simulink model "meart_host_60"  (Simulink 6.5)
settings: Solver=FixedStepDiscrete  StartTime=0.0  StopTime=Inf  RelTol=1e-3
values from neighbouring files (symbols this model uses):
  threshold = -10*std(data)    [setthresh.m]
libraries: simulink x9, xpclib x5, dspindex x4, dspsigops x2, dspstat3 x1
settings Model: Creator=adowd  LastModifiedBy=avnerw
settings OptimizationCC: InlineInvariantSignals=on
settings DebuggingCC: MultiTaskDSMMsg=warning  MultiTaskCondExecSysMsg=none  StrictBusMsg=None
settings RTWCC: IncludeERTFirstTime=on

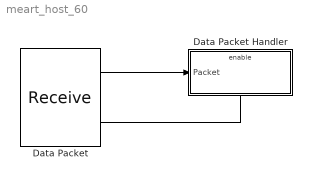
== system meart_host_60 ==
  Data Packet : xpclib/UDP/Receive  ipAddress=192.168.0.10  ipPort=25000  width=5524  sampletime=0.0008
  Data Packet Handler : Subsystem  TreatAsAtomicUnit=on
  wires:
  Data Packet/1 -> Data Packet Handler/1(Packet)
  Data Packet/2 -> Data Packet Handler/Enable

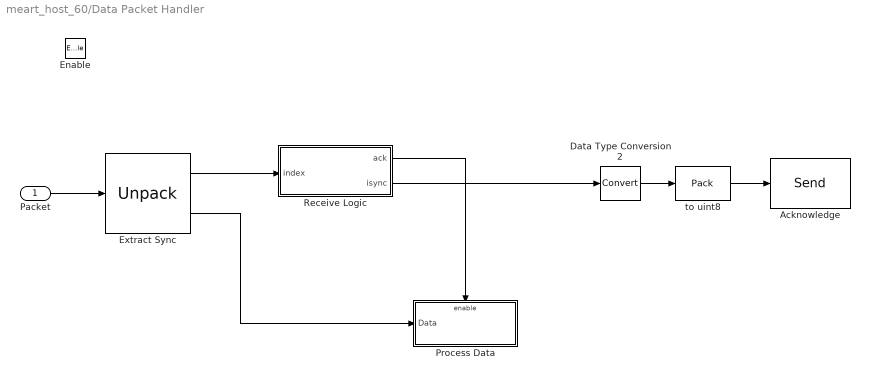
== system meart_host_60/Data Packet Handler ==
  Packet : Inport
  Enable : EnablePort
  Acknowledge : xpclib/UDP/Send  ipAddress=192.168.0.10  ipPort=25001  localPort=-1  sampletime=-1
  Data Type Conversion2 : DataTypeConversion  OutDataTypeMode=uint32
  Extract Sync : xpclib/UDP/Unpack  dimensions={1,5520}  datatypes={'uint32','uint8'}  byteAlign=1
  Process Data : Subsystem  TreatAsAtomicUnit=on
  Receive Logic : Stateflow chart
  to uint8 : xpclib/UDP/Pack  datatypes={'uint32'}  byteAlign=1
  wires:
  to uint8/1 -> Acknowledge/1
  Data Type Conversion2/1 -> to uint8/1
  Receive Logic/1(ack) -> Process Data/Enable
  Receive Logic/2(isync) -> Data Type Conversion2/1
  Extract Sync/1 -> Receive Logic/1(index)
  Extract Sync/2 -> Process Data/1(Data)
  Packet/1 -> Extract Sync/1

== system meart_host_60/Data Packet Handler/Process Data ==
  Data : Inport
  Enable : EnablePort
  Iterate Frames : Subsystem  TreatAsAtomicUnit=on
  Reshape : Reshape  OutputDimensionality=Customize (N-D)  OutputDimensions=[552,10]
  wires:
  Data/1 -> Reshape/1
  Reshape/1 -> Iterate Frames/1(Data Packet)

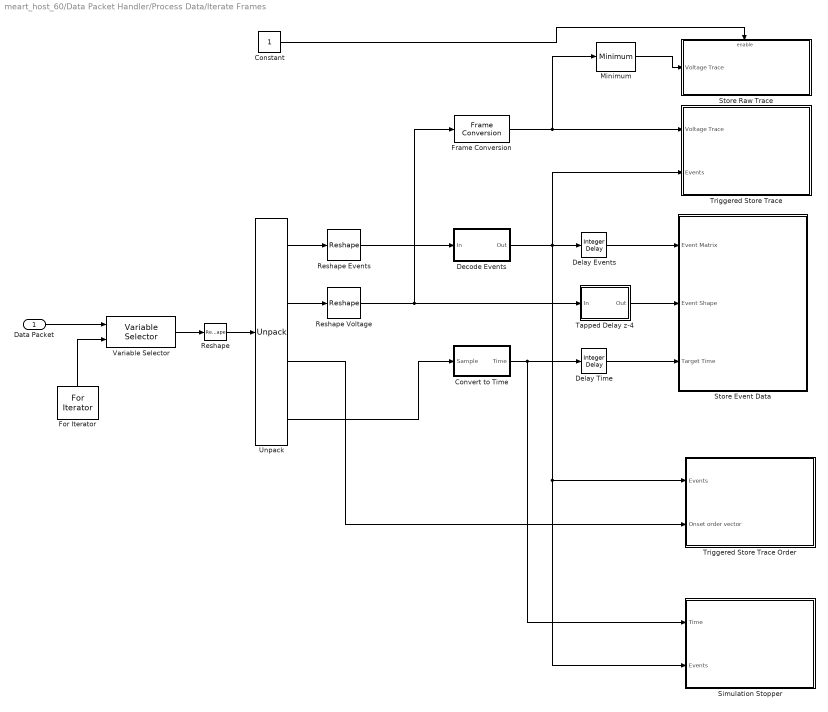
== system meart_host_60/Data Packet Handler/Process Data/Iterate Frames ==
  Data Packet : Inport
  Constant : Constant  Value=1  OutDataType=sfix(16)  ConRadixGroup=Use specified scaling  OutScaling=2^0  SampleTime=inf  FramePeriod=inf
  Convert to Time : Subsystem  mask{frametime=0.0005}
      mask prompts: frametime "Frametime (s):"
  Decode Events : Subsystem
  Delay Events : simulink/Discrete/Integer Delay  vinit=0  samptime=-1  NumDelays=3
  Delay Time : simulink/Discrete/Integer Delay  vinit=0  samptime=-1  NumDelays=3
  For Iterator : ForIterator  Orientation=up  IterationLimit=10  IterationVariableDataType=int16
  Frame Conversion : FrameConversion
  Minimum : dspstat3/Minimum  DialogController=dspfixptddg.MinMax  DialogControllerArgs=DataTag0  fcn=Value  reset=None  indexBase=One  operateOver=Each column  colComp=on  operation=minimum  roundingMode=Floor  overflowMode=off
  Reshape : Reshape
  Reshape Events : Reshape  OutputDimensionality=Customize (N-D)  OutputDimensions=[1,2]
  Reshape Voltage : Reshape  OutputDimensionality=Customize (N-D)  OutputDimensions=[8,60]
  Simulation Stopper : Subsystem  TreatAsAtomicUnit=on  mask{maxtrigs=10000, triggerchannel=61, delayframes=15*2}
      mask prompts: maxtrigs "Maximum number of triggers to concatenate:"; triggerchannel "Trigger to Channel:"; delayframes "Number of frames to delay before stopping the hosr after last trig"
  Store Event Data : Subsystem  TreatAsAtomicUnit=on
  Store Raw Trace : Subsystem  TreatAsAtomicUnit=on  mask{maxsamples=2000*3}
      mask prompts: maxsamples "Maximum number of samples  to concatenate:"
  Tapped Delay z-4 : Subsystem
  Triggered Store Trace : Subsystem  TreatAsAtomicUnit=on  mask{presamples=0, postsamples=15*2, maxrecords=3600, triggerchannel=61}
      mask prompts: presamples "Presamples (frames):"; postsamples "Postsamples (frames):"; maxrecords "Maximum number of records to concatenate:"; triggerchannel "Trigger to Channel:"
  Triggered Store Trace Order : Subsystem  TreatAsAtomicUnit=on  mask{offsettimeframes=15*2, maxrecords=10000, triggerchannel=61}
      mask prompts: offsettimeframes "offset time (frames):"; maxrecords "Maximum number of records to concatenate:"; triggerchannel "Trigger to Channel:"
  Unpack : xpclib/UDP/Unpack  dimensions={2, 480,60, 1}  datatypes={'uint32', 'int8', 'uint8','uint32'}  byteAlign=1
  Variable Selector : dspindex/Variable Selector  NumInputs=1  rowsOrCols=Columns  IdxMode=Variable  Elements=[1 3]  ZerOneIdxMode=One-based  errmode=Generate Error  FillMode=off  FillValues=0
  wires:
  Unpack/2 -> Reshape Voltage/1
  Unpack/1 -> Reshape Events/1
  Reshape Events/1 -> Decode Events/1(In)
  Decode Events/1(Out) -> Triggered Store Trace/2(Events), Delay Events/1, Triggered Store Trace Order/1(Events), Simulation Stopper/2(Events)
  Reshape Voltage/1 -> Frame Conversion/1, Tapped Delay z-4/1(In)
  Data Packet/1 -> Variable Selector/1
  For Iterator/1 -> Variable Selector/2
  Variable Selector/1 -> Reshape/1
  Reshape/1 -> Unpack/1
  Frame Conversion/1 -> Triggered Store Trace/1(Voltage Trace), Minimum/1
  Minimum/1 -> Store Raw Trace/1(Voltage Trace)
  Convert to Time/1(Time) -> Delay Time/1, Simulation Stopper/1(Time)
  Delay Time/1 -> Store Event Data/3(Target Time)
  Delay Events/1 -> Store Event Data/1(Event Matrix)
  Tapped Delay z-4/1(Out) -> Store Event Data/2(Event Shape)
  Constant/1 -> Store Raw Trace/Enable
  Unpack/4 -> Convert to Time/1(Sample)
  Unpack/3 -> Triggered Store Trace Order/2(Onset order vector)

== system meart_host_60/Data Packet Handler/Process Data/Iterate Frames/Convert to Time ==
  Sample : Inport
  Convert Seconds : Product  Inputs=**  OutDataTypeMode=double  OutScaling=2^-10
  Frametime : Constant  Orientation=up  Value=frametime  OutDataTypeMode=double  OutDataType=sfix(16)  ConRadixGroup=Use specified scaling  OutScaling=2^0  SampleTime=inf  FramePeriod=inf
  Time : Outport
  wires:
  Convert Seconds/1 -> Time/1
  Frametime/1 -> Convert Seconds/2
  Sample/1 -> Convert Seconds/1

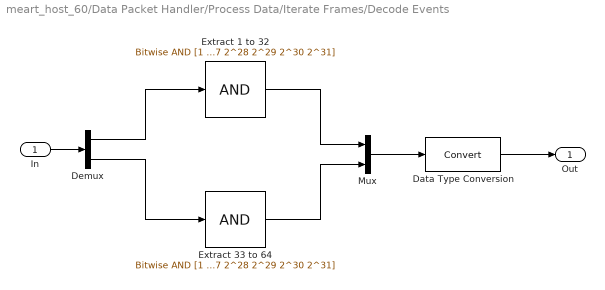
== system meart_host_60/Data Packet Handler/Process Data/Iterate Frames/Decode Events ==
  In : Inport  PortDimensions=2  DataType=uint32
  Data Type Conversion : DataTypeConversion  OutDataTypeMode=boolean
  Demux : Demux  Outputs=2
  Extract 1 to 32 : simulink/Logic and Bit Operations/Bitwise Operator  logicop=AND  UseBitMask=on  BitMask=[1 2 2^2 2^3 2^4 2^5 2^6 2^7 2^8 2^9 2^10 2^11 2^12 2^13 2^14 2^15 2^16 2^17 2^18 2^19 2^20 2^21 2^22 2^23 2^24 2^25 2^26 2^27 2^28 2^29 2^30 2^31]  BitMaskRealWorld=Stored Integer
  Extract 33 to 64 : simulink/Logic and Bit Operations/Bitwise Operator  logicop=AND  UseBitMask=on  BitMask=[1 2 2^2 2^3 2^4 2^5 2^6 2^7 2^8 2^9 2^10 2^11 2^12 2^13 2^14 2^15 2^16 2^17 2^18 2^19 2^20 2^21 2^22 2^23 2^24 2^25 2^26 2^27 2^28 2^29 2^30 2^31]  BitMaskRealWorld=Stored Integer
  Mux : Mux  Inputs=2
  Out : Outport  DataType=boolean
  wires:
  In/1 -> Demux/1
  Demux/1 -> Extract 1 to 32/1
  Demux/2 -> Extract 33 to 64/1
  Extract 33 to 64/1 -> Mux/2
  Mux/1 -> Data Type Conversion/1
  Data Type Conversion/1 -> Out/1
  Extract 1 to 32/1 -> Mux/1

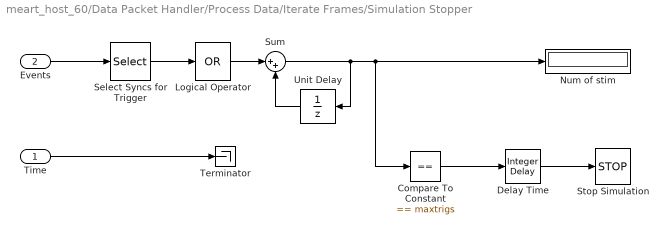
== system meart_host_60/Data Packet Handler/Process Data/Iterate Frames/Simulation Stopper ==
  Time : Inport
  Events : Inport  Port=2
  Compare To Constant : simulink/Logic and Bit Operations/Compare To Constant  SystemSampleTime=-1  relop===  const=maxtrigs  LogicOutDataTypeMode=boolean  ZeroCross=off
  Delay Time : simulink/Discrete/Integer Delay  vinit=0  samptime=-1  NumDelays=delayframes
  Logical Operator : Logic  Operator=OR  Inputs=1  AllPortsSameDT=off  OutDataTypeMode=Boolean
  Num of stim : Display
  Select Syncs for Trigger : Selector  InputType=Vector  ElementSrc=Internal  Elements=triggerchannel  RowSrc=Internal  Rows=1  ColumnSrc=Internal  Columns=1  InputPortWidth=64  IndexIsStartValue=off
  Stop Simulation : Stop
  Sum : Sum  Inputs=|++  OutDataTypeMode=double
  Terminator : Terminator
  Unit Delay : UnitDelay  Orientation=left  SampleTime=-1
  wires:
  Time/1 -> Terminator/1
  Select Syncs for Trigger/1 -> Logical Operator/1
  Events/1 -> Select Syncs for Trigger/1
  Sum/1 -> Compare To Constant/1, Num of stim/1, Unit Delay/1
  Compare To Constant/1 -> Delay Time/1
  Unit Delay/1 -> Sum/2
  Logical Operator/1 -> Sum/1
  Delay Time/1 -> Stop Simulation/1

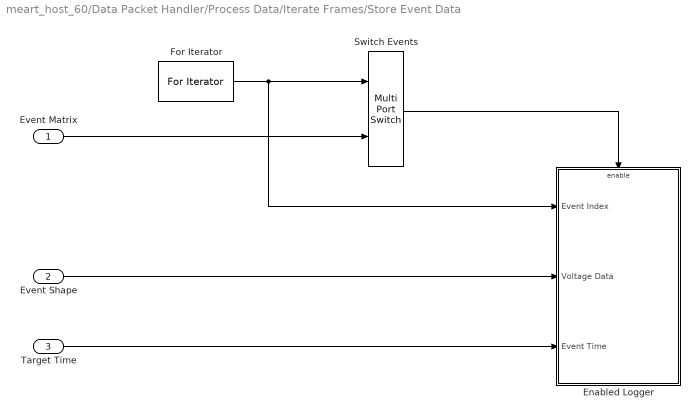
== system meart_host_60/Data Packet Handler/Process Data/Iterate Frames/Store Event Data ==
  Event Matrix : Inport  PortDimensions=64
  Event Shape : Inport  Port=2
  Target Time : Inport  Port=3  DataType=double
  Enabled Logger : Subsystem  TreatAsAtomicUnit=on
  For Iterator : ForIterator  IterationLimit=64  IterationVariableDataType=int8
  Switch Events : MultiPortSwitch  Inputs=1  SaturateOnIntegerOverflow=on  InputSameDT=on
  wires:
  Target Time/1 -> Enabled Logger/3(Event Time)
  Switch Events/1 -> Enabled Logger/Enable
  Event Matrix/1 -> Switch Events/2
  For Iterator/1 -> Switch Events/1, Enabled Logger/1(Event Index)
  Event Shape/1 -> Enabled Logger/2(Voltage Data)

== system meart_host_60/Data Packet Handler/Process Data/Iterate Frames/Store Raw Trace ==
  Voltage Trace : Inport
  Enable : EnablePort
  Raw Trace  to Workspace : ToWorkspace  VariableName=datalog_rawtrace  SampleTime=-1  SaveFormat=Array
      settings: MaxDataPoints=maxsamples
  wires:
  Voltage Trace/1 -> Raw Trace  to Workspace/1

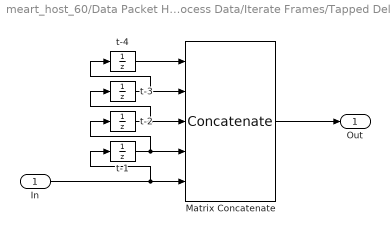
== system meart_host_60/Data Packet Handler/Process Data/Iterate Frames/Tapped Delay z-4 ==
  In : Inport
  Matrix Concatenate : Concatenate  NumInputs=5  Mode=Vertical matrix concatenation
  t-{1..4} (4 alike) : UnitDelay  SampleTime=-1
  Out : Outport
  wires:
  In/1 -> Matrix Concatenate/5, t-1/1
  t-1/1 -> Matrix Concatenate/4, t-2/1
  t-2/1 -> Matrix Concatenate/3, t-3/1
  t-3/1 -> t-4/1, Matrix Concatenate/2
  t-4/1 -> Matrix Concatenate/1
  Matrix Concatenate/1 -> Out/1

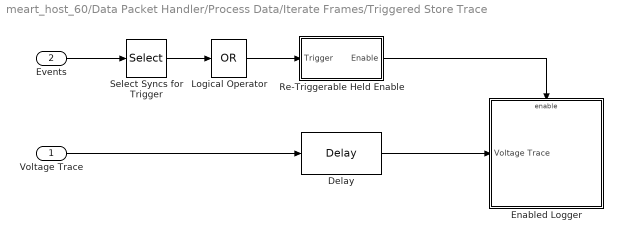
== system meart_host_60/Data Packet Handler/Process Data/Iterate Frames/Triggered Store Trace ==
  Voltage Trace : Inport
  Events : Inport  Port=2
  Delay : dspsigops/Delay  dly_unit=Samples  delay=presamples*8  ic_detail=off  dif_ic_for_ch=off  dif_ic_for_dly=off  ic=0  reset_popup=None
  Enabled Logger : Subsystem  TreatAsAtomicUnit=on
  Logical Operator : Logic  Operator=OR  Inputs=1  AllPortsSameDT=off  OutDataTypeMode=Boolean
  Re-Triggerable Held Enable : Subsystem  mask{holdtimesamples=presamples + postsamples}
      mask prompts: holdtimesamples "Hold time (samples)"
      mask Display:
      | plot([.1 .2 .2 .2 .3 .3 .3 .4], [.1 .1 .9 .1 .1 .9 .1 .1 ])
      | plot([.4 .8 .8 .9], [.9 .9 .1 .1])
      | plot([.4 .7 .65 .7 .65], [.35 .35 .40 .35 .30])
      | text(0.5, 0.6, num2str(holdtimesamples))
  Select Syncs for Trigger : Selector  InputType=Vector  ElementSrc=Internal  Elements=triggerchannel  RowSrc=Internal  Rows=1  ColumnSrc=Internal  Columns=1  InputPortWidth=64  IndexIsStartValue=off
  wires:
  Voltage Trace/1 -> Delay/1
  Re-Triggerable Held Enable/1(Enable) -> Enabled Logger/Enable
  Delay/1 -> Enabled Logger/1(Voltage Trace)
  Select Syncs for Trigger/1 -> Logical Operator/1
  Logical Operator/1 -> Re-Triggerable Held Enable/1(Trigger)
  Events/1 -> Select Syncs for Trigger/1

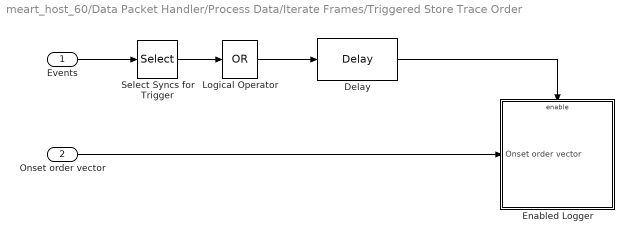
== system meart_host_60/Data Packet Handler/Process Data/Iterate Frames/Triggered Store Trace Order ==
  Events : Inport
  Onset order vector : Inport  Port=2
  Delay : dspsigops/Delay  dly_unit=Samples  delay=offsettimeframes  ic_detail=off  dif_ic_for_ch=off  dif_ic_for_dly=off  ic=0  reset_popup=None
  Enabled Logger : Subsystem  TreatAsAtomicUnit=on
  Logical Operator : Logic  Operator=OR  Inputs=1  AllPortsSameDT=off  OutDataTypeMode=Boolean
  Select Syncs for Trigger : Selector  InputType=Vector  ElementSrc=Internal  Elements=triggerchannel  RowSrc=Internal  Rows=1  ColumnSrc=Internal  Columns=1  InputPortWidth=64  IndexIsStartValue=off
  wires:
  Events/1 -> Select Syncs for Trigger/1
  Logical Operator/1 -> Delay/1
  Select Syncs for Trigger/1 -> Logical Operator/1
  Delay/1 -> Enabled Logger/Enable
  Onset order vector/1 -> Enabled Logger/1(Onset order vector)

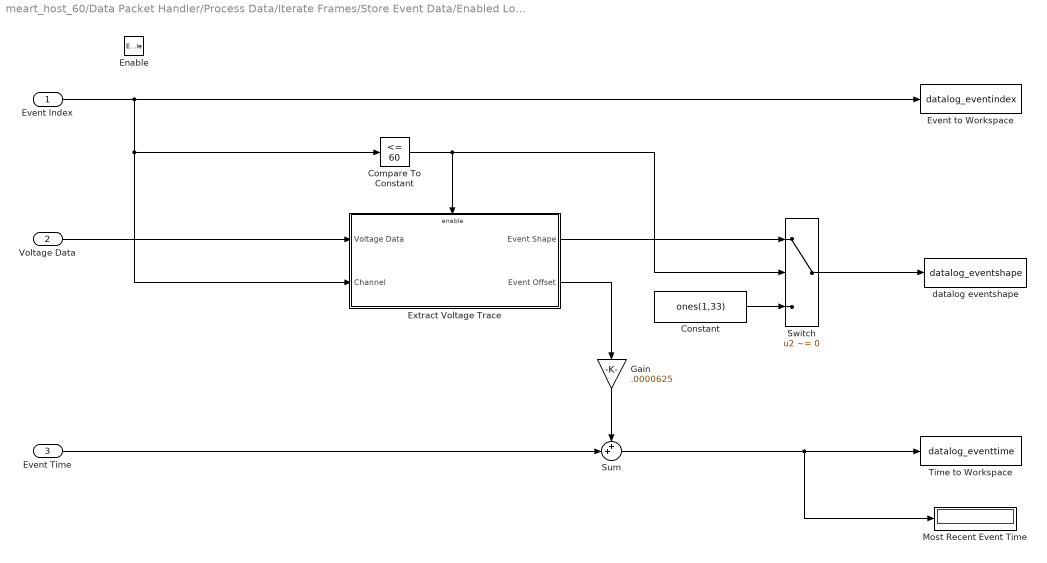
== system meart_host_60/Data Packet Handler/Process Data/Iterate Frames/Store Event Data/Enabled Logger ==
  Event Index : Inport
  Voltage Data : Inport  Port=2
  Event Time : Inport  Port=3
  Enable : EnablePort
  Compare To Constant : simulink/Logic and Bit Operations/Compare To Constant  SystemSampleTime=-1  relop=<=  const=60  LogicOutDataTypeMode=uint8  ZeroCross=off
  Constant : Constant  Value=ones(1,33)  OutDataTypeMode=int8  OutDataType=sfix(16)  ConRadixGroup=Use specified scaling  OutScaling=2^0  SampleTime=inf  FramePeriod=inf
  Event to Workspace : ToWorkspace  VariableName=datalog_eventindex  SampleTime=-1  SaveFormat=Array
  Extract Voltage Trace : Subsystem
  Gain : Gain  Orientation=down  Gain=.0000625  ParameterDataTypeMode=Specify via dialog  ParameterDataType=float('double')
  Most Recent Event Time : Display
  Sum : Sum  Inputs=++|
  Switch : Switch  Criteria=u2 ~= 0  ZeroCross=off
  Time to Workspace : ToWorkspace  VariableName=datalog_eventtime  SampleTime=-1  SaveFormat=Array
  datalog eventshape : ToWorkspace  VariableName=datalog_eventshape  SampleTime=-1  SaveFormat=Array
  wires:
  Event Index/1 -> Extract Voltage Trace/2(Channel), Compare To Constant/1, Event to Workspace/1
  Voltage Data/1 -> Extract Voltage Trace/1(Voltage Data)
  Compare To Constant/1 -> Extract Voltage Trace/Enable, Switch/2
  Switch/1 -> datalog eventshape/1
  Extract Voltage Trace/1(Event Shape) -> Switch/1
  Constant/1 -> Switch/3
  Sum/1 -> Most Recent Event Time/1, Time to Workspace/1
  Event Time/1 -> Sum/2
  Extract Voltage Trace/2(Event Offset) -> Gain/1
  Gain/1 -> Sum/1

== system meart_host_60/Data Packet Handler/Process Data/Iterate Frames/Triggered Store Trace/Enabled Logger ==
  Voltage Trace : Inport
  Enable : EnablePort
  Trace  to Workspace : ToWorkspace  VariableName=datalog_trigtrace  SampleTime=-1  SaveFormat=Array
      settings: MaxDataPoints="maxrecords *  (presamples+postsamples) * 8"
  wires:
  Voltage Trace/1 -> Trace  to Workspace/1

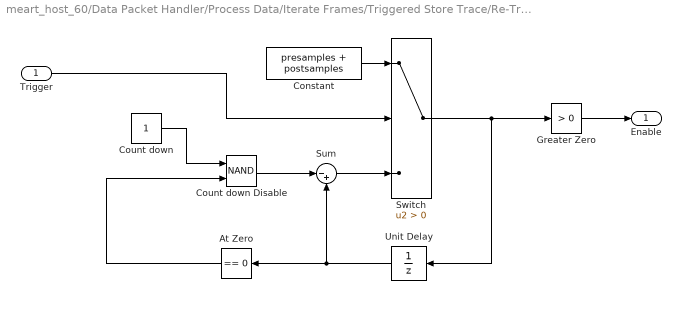
== system meart_host_60/Data Packet Handler/Process Data/Iterate Frames/Triggered Store Trace/Re-Triggerable Held Enable ==
  Trigger : Inport  DataType=boolean
  At Zero : simulink/Logic and Bit Operations/Compare To Zero  Orientation=left  SystemSampleTime=-1  relop===  LogicOutDataTypeMode=boolean  ZeroCross=off
  Constant : Constant  Value=presamples + postsamples  OutDataTypeMode=uint32  OutDataType=sfix(16)  ConRadixGroup=Use specified scaling  OutScaling=2^0  SampleTime=inf  FramePeriod=inf
  Count down : Constant  Value=1  OutDataTypeMode=boolean  OutDataType=sfix(16)  ConRadixGroup=Use specified scaling  OutScaling=2^0  SampleTime=inf  FramePeriod=inf
  Count down Disable : Logic  Operator=NAND  AllPortsSameDT=off  OutDataTypeMode=Specify via dialog
  Greater Zero : simulink/Logic and Bit Operations/Compare To Zero  SystemSampleTime=-1  relop=>  LogicOutDataTypeMode=boolean  ZeroCross=off
  Sum : Sum  Inputs=|-+  OutDataTypeMode=uint32
  Switch : Switch  Criteria=u2 > Threshold
  Unit Delay : UnitDelay  Orientation=left  SampleTime=-1
  Enable : Outport
  wires:
  Constant/1 -> Switch/1
  Switch/1 -> Greater Zero/1, Unit Delay/1
  Unit Delay/1 -> At Zero/1, Sum/2
  At Zero/1 -> Count down Disable/2
  Sum/1 -> Switch/3
  Count down Disable/1 -> Sum/1
  Count down/1 -> Count down Disable/1
  Trigger/1 -> Switch/2
  Greater Zero/1 -> Enable/1

== system meart_host_60/Data Packet Handler/Process Data/Iterate Frames/Triggered Store Trace Order/Enabled Logger ==
  Onset order vector : Inport
  Enable : EnablePort
  Trace  to Workspace : ToWorkspace  VariableName=datalog_onsetorder  SampleTime=-1  SaveFormat=Array
      settings: MaxDataPoints=maxrecords
  wires:
  Onset order vector/1 -> Trace  to Workspace/1

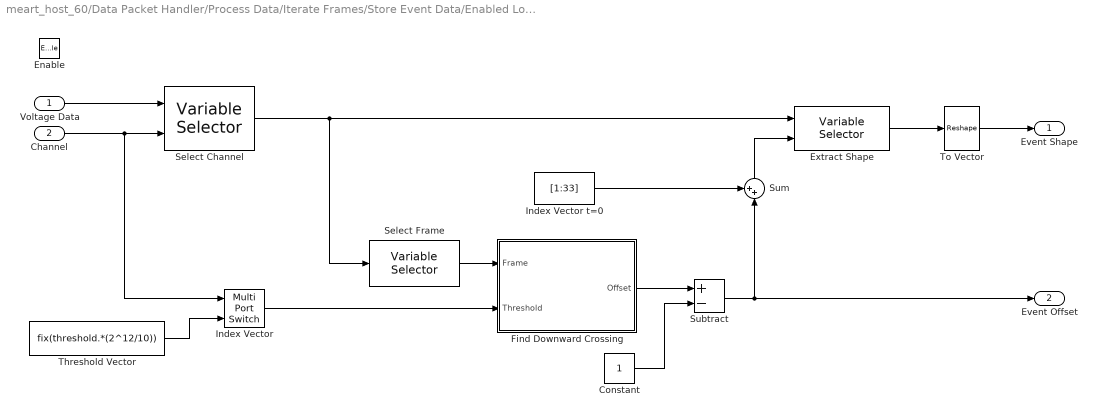
== system meart_host_60/Data Packet Handler/Process Data/Iterate Frames/Store Event Data/Enabled Logger/Extract Voltage Trace ==
  Voltage Data : Inport
  Channel : Inport  Port=2
  Enable : EnablePort
  Constant : Constant  Value=1  OutDataTypeMode=uint8  OutDataType=sfix(16)  ConRadixGroup=Use specified scaling  OutScaling=2^0  SampleTime=inf  FramePeriod=inf
  Extract Shape : dspindex/Variable Selector  NumInputs=1  rowsOrCols=Rows  IdxMode=Variable  Elements=[1 3]  ZerOneIdxMode=One-based  errmode=Generate Error  FillMode=on  FillValues=0
  Find Downward Crossing : Subsystem  TreatAsAtomicUnit=on
  Index Vector : MultiPortSwitch  Inputs=1
  Index Vector t=0 : Constant  Value=[1:33]  OutDataTypeMode=uint8  OutDataType=sfix(16)  ConRadixGroup=Use specified scaling  OutScaling=2^0  SampleTime=inf  FramePeriod=inf
  Select Channel : dspindex/Variable Selector  NumInputs=1  rowsOrCols=Columns  IdxMode=Variable  Elements=[1 3]  ZerOneIdxMode=One-based  errmode=Generate Error  FillMode=off  FillValues=0
  Select Frame : dspindex/Variable Selector  NumInputs=1  rowsOrCols=Rows  IdxMode=Fixed  Elements=9:16  ZerOneIdxMode=One-based  errmode=Generate Error  FillMode=off  FillValues=0
  Subtract : Sum  Inputs=+-  OutDataTypeMode=uint8  OutScaling=2^-10
  Sum : Sum  Orientation=up  Inputs=++|  OutDataTypeMode=uint8
  Threshold Vector : Constant  Value=fix(threshold.*(2^12/10))  OutDataType=sfix(16)  ConRadixGroup=Use specified scaling  OutScaling=2^0  SampleTime=inf  FramePeriod=inf
  To Vector : Reshape
  Event Shape : Outport
  Event Offset : Outport  Port=2  OutputWhenDisabled=reset  InitialOutput=0
  wires:
  Channel/1 -> Select Channel/2, Index Vector/1
  Voltage Data/1 -> Select Channel/1
  To Vector/1 -> Event Shape/1
  Select Frame/1 -> Find Downward Crossing/1(Frame)
  Index Vector t=0/1 -> Sum/1
  Sum/1 -> Extract Shape/2
  Extract Shape/1 -> To Vector/1
  Find Downward Crossing/1(Offset) -> Subtract/1
  Threshold Vector/1 -> Index Vector/2
  Select Channel/1 -> Extract Shape/1, Select Frame/1
  Index Vector/1 -> Find Downward Crossing/2(Threshold)
  Subtract/1 -> Sum/2, Event Offset/1
  Constant/1 -> Subtract/2

== system meart_host_60/Data Packet Handler/Process Data/Iterate Frames/Store Event Data/Enabled Logger/Extract Voltage Trace/Find Downward Crossing ==
  Frame : Inport
  Threshold : Inport  Port=2
  Index Vector : MultiPortSwitch  Inputs=1
  Relational Operator : RelationalOperator  LogicOutDataTypeMode=Boolean
  While Iterator : WhileIterator  MaxIters=8  WhileBlockType=do-while  ResetStates=reset  ShowIterationPort=on  OutputDataType=int8
  Offset : Outport
  wires:
  Relational Operator/1 -> While Iterator/1
  While Iterator/1 -> Offset/1, Index Vector/1
  Frame/1 -> Index Vector/2
  Index Vector/1 -> Relational Operator/1
  Threshold/1 -> Relational Operator/2

== matlab function Data Packet Handler/Receive Logic ==
  data: index input inherited; ack output inherited; isync output inherited
function [ack,isync] = rxsync(index)
% Receive Synchronization logic - State controller for the Host application 
%   that receives a stream of data from the target
%
%  The index is the sync value that was attached to the recently 
%  received packet. If the index is the next integer in the sync sequenc, 
%  then we should save the data and then increment the sequency to watch 
%  for the
%  next packet.  Otherwise, if the received index is not the next value 
%  in the sequence, toss out the data (i.e. don't save it) and retransmit to 
%  the sync value of the last accepted packet. This is necessary to avoid 
%  a deadlock caused by a lost response.  
%  
persistent sync;
if isempty(sync)
    % First time, everything is good!  
    sync = index;
    ack = 1;
else
    if index == sync+1,
        sync = index;
        ack = 1;
    else
        ack = 0;
    end
end
isync = sync;
return;
